simulink model "Two_mass_sim"  (R2024a)
settings: Solver=VariableStepAuto  StartTime=0.0  StopTime=10.0  FixedStep=0.001  RelTol=1e-3
values from neighbouring files (symbols this model uses):
  C12 = zeta*(2*sqrt(meff*K12))    [two_mass_system.m]
  J1 = 0.195e-3    (= 0.000195)    [two_mass_system.m]
  J2 = (omega_r^2*J1/omega_ar^2) - J1    (= 4.095e-05)    [two_mass_system.m]
  Jm = J1    (= 0.000195)    [two_mass_system.m]
  K12 = omega_ar^2 * J2    (= 404.160300225)    [two_mass_system.m]
  KPP = BW * 0.5 * pi    (= 157.079632679)    [two_mass_system.m]
  KVP = BW * 2 * pi    (= 628.318530718)    [two_mass_system.m]
settings Model: Creator=KATE.HUNG  LastModifiedBy=VSCLAB-3060
settings SolverCC: AlgebraicLoopSolver=TrustRegion
settings DebuggingCC: UnconnectedInputMsg=warning  UnconnectedOutputMsg=warning  UnconnectedLineMsg=warning
settings ModelReferenceCC: EnableRefExpFcnMdlSchedulingChecks=on
settings RTWCC: GPUComputeCapability=3.5

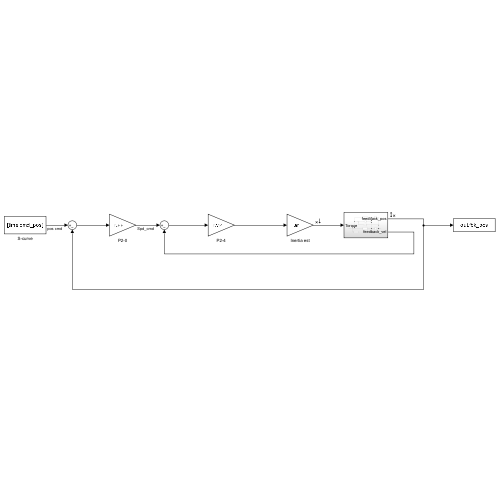
[thumbnail: Simulink's stored preview of the top-level diagram]
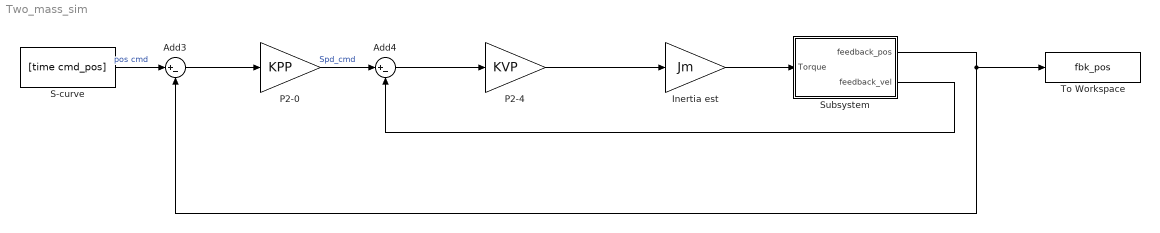
== system Two_mass_sim ==
  Add3 : Sum  Inputs=|+-
  Add4 : Sum  Inputs=|+-
  Inertia est : Gain  Gain=Jm
  P2-0 : Gain  Gain=KPP
  P2-4 : Gain  Gain=KVP
  S-curve : FromWorkspace  VariableName=[time cmd_pos]
  Subsystem : Subsystem
  To Workspace : ToWorkspace  VariableName=fbk_pos  SaveFormat=Timeseries  SampleTime=-1
  wires:
  Add3/1 -> P2-0/1
  P2-4/1 -> Inertia est/1
  Add4/1 -> P2-4/1
  P2-0/1 -> Add4/1  "Spd_cmd"
  S-curve/1 -> Add3/1  "pos cmd"
  Subsystem/1(feedback_pos) -> To Workspace/1, Add3/2
  Inertia est/1 -> Subsystem/1(Torque)
  Subsystem/2(feedback_vel) -> Add4/2

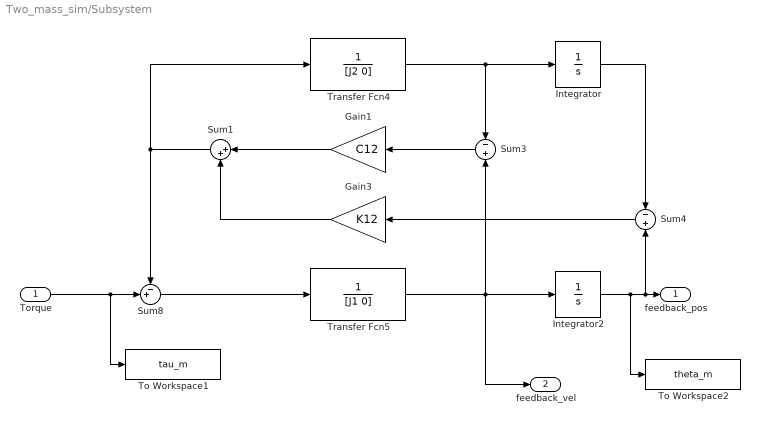
== system Two_mass_sim/Subsystem ==
  Torque : Inport
  Gain1 : Gain  Gain=C12
  Gain3 : Gain  Gain=K12
  Integrator : Integrator
  Integrator2 : Integrator
  Sum1 : Sum  Inputs=|++
  Sum3 : Sum  Inputs=-|+
  Sum4 : Sum  Inputs=-|+
  Sum8 : Sum  Inputs=-+|
  To Workspace1 : ToWorkspace  VariableName=tau_m  SaveFormat=Timeseries  SampleTime=-1
  To Workspace2 : ToWorkspace  VariableName=theta_m  SaveFormat=Timeseries  SampleTime=-1
  Transfer Fcn4 : TransferFcn  Denominator=[J2 0]
  Transfer Fcn5 : TransferFcn  Denominator=[J1 0]
  feedback_pos : Outport
  feedback_vel : Outport  Port=2
  wires:
  Gain1/1 -> Sum1/1
  Sum4/1 -> Gain3/1
  Transfer Fcn4/1 -> Sum3/1, Integrator/1
  Sum3/1 -> Gain1/1
  Sum8/1 -> Transfer Fcn5/1
  Gain3/1 -> Sum1/2
  Transfer Fcn5/1 -> Sum3/2, feedback_vel/1, Integrator2/1
  Sum1/1 -> Transfer Fcn4/1, Sum8/1
  Integrator/1 -> Sum4/1
  Integrator2/1 -> To Workspace2/1, Sum4/2, feedback_pos/1
  Torque/1 -> To Workspace1/1, Sum8/2
